simulink model "untitled"  (R2017b)
settings: Solver=VariableStepAuto  StartTime=0.0  StopTime=10.0  RelTol=1e-3
undefined symbols (not defined in the file): b_contact_RW, C_F_alpha, C_F_kappa, Cylinder, Dtheta0, epsilon, g, k_contact_RW, lengthRW, massRW, Parts_Lib, radiusRW, sigma, v0, X, xPla, Y, yPla, Z, zPla
libraries: nesl_utility x20, sm_lib x11, vrlib x6
settings Model: Creator=r_ahmed_afzal  LastModifiedBy=r_ahmed_afzal

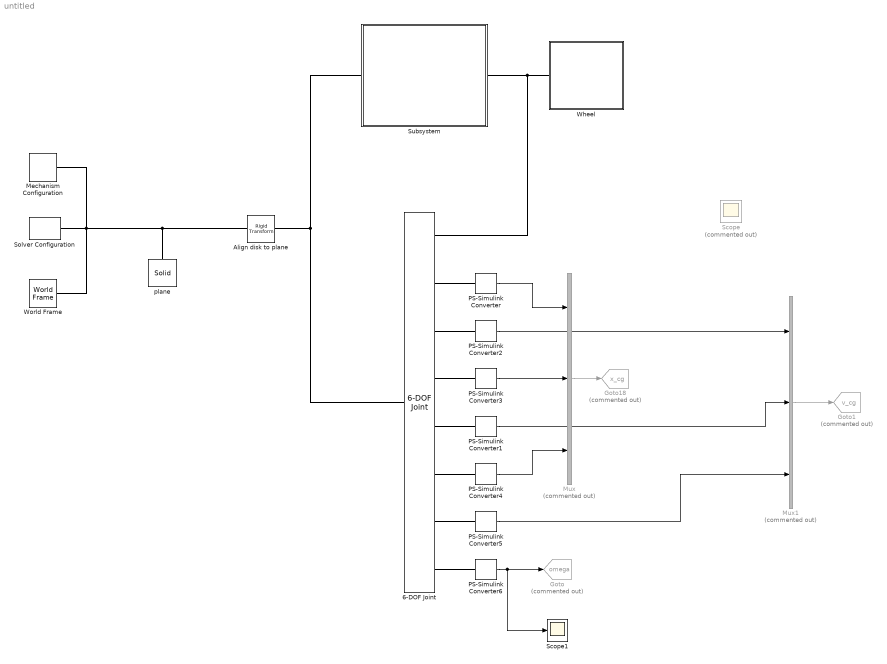
== system untitled ==
  6-DOF Joint : sm_lib/Joints/6-DOF Joint  SenseConstraintForce=off  SenseConstraintForceX=off  SenseConstraintForceY=off  SenseConstraintForceZ=off  SenseConstraintTorque=off  SenseConstraintTorqueX=off  SenseConstraintTorqueY=off  SenseConstraintTorqueZ=off  SenseTotalForce=off  SenseTotalForceX=off  SenseTotalForceY=off  SenseTotalForceZ=off  SenseTotalTorque=off  SenseTotalTorqueX=off  SenseTotalTorqueY=off  SenseTotalTorqueZ=off  CompositeWrenchDir=FollowerOnBase  CompositeWrenchFrame=BaseFrame  PxEquilibriumPosition=0  PxEquilibriumPositionUnits=m  PxSpringStiffness=0  PxSpringStiffnessUnits=N/m  PxDampingCoefficient=0  PxDampingCoefficientUnits=N/(m/s)  PxTorqueActuationMode=NoTorque  PxMotionActuationMode=ComputedMotion  PxSensePosition=on  PxSenseVelocity=on  PxSenseAcceleration=off  PxSenseTorqueForce=off  PxPositionTargetSpecify=on  PxPositionTargetPriority=High  PxPositionTargetValue=-xPla/2 + 0.1  PxPositionTargetValueUnits=m  PxVelocityTargetSpecify=off  PxVelocityTargetPriority=High  PxVelocityTargetValue=0  PxVelocityTargetValueUnits=m/s  PyEquilibriumPosition=0  PyEquilibriumPositionUnits=m  PySpringStiffness=0  PySpringStiffnessUnits=N/m  PyDampingCoefficient=0  PyDampingCoefficientUnits=N/(m/s)  PyTorqueActuationMode=NoTorque  PyMotionActuationMode=ComputedMotion  PySensePosition=on  PySenseVelocity=on  PySenseAcceleration=off  PySenseTorqueForce=off  PyPositionTargetSpecify=on  PyPositionTargetPriority=High  PyPositionTargetValue=radiusRW  PyPositionTargetValueUnits=m  PyVelocityTargetSpecify=off  PyVelocityTargetPriority=High  PyVelocityTargetValue=0  PyVelocityTargetValueUnits=m/s  PzEquilibriumPosition=0  PzEquilibriumPositionUnits=m  PzSpringStiffness=0  PzSpringStiffnessUnits=N/m  PzDampingCoefficient=0  PzDampingCoefficientUnits=N/(m/s)  PzTorqueActuationMode=NoTorque  PzMotionActuationMode=ComputedMotion  PzSensePosition=on  PzSenseVelocity=on  PzSenseAcceleration=off  PzSenseTorqueForce=off  PzPositionTargetSpecify=off  PzPositionTargetPriority=High  PzPositionTargetValue=0  PzPositionTargetValueUnits=m  PzVelocityTargetSpecify=off  PzVelocityTargetPriority=High  PzVelocityTargetValue=0  PzVelocityTargetValueUnits=m/s  SphDefPosRotationMethod=None  SphDefPosRotationAngleUnits=deg  SphDefPosRotationStandardAxis=+Z  SphDefPosRotationAngle=0.0  SphDefPosRotationArbitraryAxis=[0 0 1]  SphDefPosFollAlignAxisA=+X  SphDefPosBaseAlignAxisA=+Y  SphDefPosFollAlignAxisB=+Y  SphDefPosBaseAlignAxisB=+Z  SphDefPosRotationSequenceAxes=FollowerAxes  SphDefPosRotationSequence=XYX  SphDefPosRotationSequenceAngles=[0 0 0]  SphDefPosRotationSequenceAnglesUnits=deg  SphDefPosRotationMatrix=[1 0 0; 0 1 0; 0 0 1]  SphEqPosRotationMethod=None  SphEqPosRotationAngleUnits=deg  SphEqPosRotationStandardAxis=+Z  SphEqPosRotationAngle=0.0  SphEqPosRotationArbitraryAxis=[0 0 1]  SphEqPosFollAlignAxisA=+X  SphEqPosBaseAlignAxisA=+Y  SphEqPosFollAlignAxisB=+Y  SphEqPosBaseAlignAxisB=+Z  SphEqPosRotationSequenceAxes=FollowerAxes  SphEqPosRotationSequence=XYX  SphEqPosRotationSequenceAngles=[0 0 0]  SphEqPosRotationSequenceAnglesUnits=deg  SphEqPosRotationMatrix=[1 0 0; 0 1 0; 0 0 1]  SphSpringStiffness=0  SphSpringStiffnessUnits=N*m/deg  SphDampingCoefficient=0  SphDampingCoefficientUnits=N*m/(deg/s)  SphActuateTorqueX=off  SphActuateTorqueY=off  SphActuateTorqueZ=off  SphActuateTorque=off  SphTorqueActuationMode=NoTorque  SphMotionActuationMode=ComputedMotion  SphActuationFrame=BaseFrame  SphSensePosition=off  SphSenseVelocityX=off  SphSenseVelocityY=off  SphSenseVelocityZ=off  SphSenseVelocity=on  SphSenseAccelerationX=off  SphSenseAccelerationY=off  SphSenseAccelerationZ=off  SphSenseAcceleration=off  SphSenseTorqueX=off  SphSenseTorqueY=off  SphSenseTorqueZ=off  SphSenseTorqueForce=off  SphSensingFrame=FollowerFrame  SphPositionTargetRotationMethod=None  SphPositionTargetRotationAngleUnits=deg  SphPositionTargetRotationStandardAxis=+Z  SphPositionTargetRotationAngle=0.0  SphPositionTargetRotationArbitraryAxis=[0 0 1]  SphPositionTargetFollAlignAxisA=+X  SphPositionTargetBaseAlignAxisA=+Y  SphPositionTargetFollAlignAxisB=+Y  SphPositionTargetBaseAlignAxisB=+Z  SphPositionTargetRotationSequenceAxes=FollowerAxes  SphPositionTargetRotationSequence=XYX  SphPositionTargetRotationSequenceAngles=[0 0 0]  SphPositionTargetRotationSequenceAnglesUnits=deg  SphPositionTargetRotationMatrix=[1 0 0; 0 1 0; 0 0 1]  SphPositionTargetSpecify=off  SphPositionTargetPriority=High  SphVelocityTargetValue=[0 0 Dtheta0]  SphVelocityTargetValueUnits=rad/s  SphVelocityTargetSpecify=on  SphVelocityTargetPriority=High  SphVelocityTargetInFollowerFrame=on
  Align disk to plane : sm_lib/Frames and Transforms/Rigid Transform  TranslationMethod=None  TranslationStandardOffset=0  TranslationLengthUnit=m  TranslationStandardAxis=+Z  TranslationCartesianOffset=[0 0 0]  TranslationROffset=0  TranslationROffsetUnits=m  TranslationZOffset=0  TranslationZOffsetUnits=m  TranslationThetaOffset=0  TranslationThetaOffsetUnits=deg  RotationMethod=AlignedAxes  RotationAngleUnits=deg  RotationStandardAxis=-X  RotationAngle=90  RotationArbitraryAxis=[0 0 1]  FollAlignAxisA=+Y  BaseAlignAxisA=+Z  FollAlignAxisB=+X  BaseAlignAxisB=+X  RotationSequenceAxes=FollowerAxes  RotationSequence=XYX  RotationSequenceAngles=[0 0 0]  RotationSequenceAnglesUnits=deg  RotationMatrix=[1 0 0; 0 1 0; 0 0 1]
  Goto : Goto  Commented=on  GotoTag=omega  TagVisibility=global
  Goto1 : Goto  Commented=on  GotoTag=v_cg  TagVisibility=global
  Goto18 : Goto  Commented=on  GotoTag=x_cg  TagVisibility=global
  Mechanism Configuration : sm_lib/Utilities/Mechanism Configuration  UniformGravity=Constant  GravityVector=[0 0 -g]  GravityUnits=m/s^2  LinearizationDelta=0.001
  Mux : Mux  Commented=on  Inputs=3
  Mux1 : Mux  Commented=on  Inputs=3
  PS-Simulink Converter{,1..6} (7 alike) : nesl_utility/PS-Simulink Converter  PhysicalDomain=network_engine_domain  SubClassName=ps_output  LeftPortType=input  RightPortType=output  PseudoPeriodic=off  Frequencies=[]  Unit=1  AffineConversion=off
  Scope : Scope  Commented=on
  Scope1 : Scope
  Solver Configuration : nesl_utility/Solver Configuration  PhysicalDomain=network_engine_domain  SubClassName=solver  LeftPortType=input  RightPortType=generic  Accelerate=off  Tones=[]  Harmonics=[]  SimulateNoise=off  Profile=off  UseLocalSampling=off  EnableSwitchedLinearOptims=on  FrequencyDomain=off  UseCCode=off  RelTol=0.001  AbsTol=1e-06  MinStep=1e-09  ToWorkspace=off  RevertToSquareIcSolve=off  NumHomotopyIterations=100  PhasorMode=off  PhasorModeNumHarmonics=1  DoDC=off  ResidualTolerance=1e-09  UseLocalSolver=off  LocalSolverChoice=NE_BACKWARD_EULER_ADVANCER  LocalSolverSampleTime=0.001  DoFixedCost=off  MaxNonlinIter=3  MaxModeIter=2  LinearAlgebra=Sparse  DelaysMemoryBudget=1024  AutomaticFiltering=on  FilteringTimeConstant=0.001
  Subsystem : Subsystem
  Wheel : Subsystem  Tag=CustomStyle  AncestorBlock=Parts_Lib/Cylinder  mask(Solid Cylinder with Markings){cyl_radius=radiusRW, cyl_length=lengthRW, cyl_density=1000, cyl_color=blue, cyl_opacity=1, cyl_color_custom=[0.7920    0.9900    0.9900], mark_radius=[0.75 0.5], mark_len_factor=1.01, mark_angle=60, mark_color=purple, mark_opacity=1}
      mask prompts: cyl_radius "Radius (m)"; cyl_length "Length (m)"; cyl_density "Density (kg/m^3)"; cyl_color "Color"; cyl_opacity "Opacity (0-1)"; cyl_color_custom "Custom Color (rgb)"; mark_radius "Outer, inner radius (% of cylinder radius)"; mark_len_factor "Length (factor of cylinder length)"; mark_angle "Sweep angle (deg)"; mark_color "Color"; mark_opacity "Opacity (0-1)"
      mask init:
      | curblk = gcb;
      | if strcmp(get_param(curblk,'cyl_color'),'red')
      |     set_param([curblk '/Cylinder'],'GraphicDiffuseColor','[0.8 0.0 0.2]');
      |     set_param(curblk,'BackGroundColor','[0.901961, 0.396078, 0.396078]');
      | elseif strcmp(get_param(gcb,'cyl_color'),'blue')
      |     set_param([curblk '/Cylinder'],'GraphicDiffuseColor','[0.0 0.5 0.7]');
      |     set_param(curblk,'BackGroundColor','[0.541176, 0.698039, 0.901961]');
      | elseif strcmp(get_param(gcb,'cyl_color'),'yellow')
      |     set_param([curblk '/Cylinder'],'GraphicDiffuseColor','[1.0 1.0 0.0]');
      |     set_param(curblk,'BackGroundColor','[0.905882, 0.890196, 0.392157]');
      | elseif strcmp(get_param(gcb,'cyl_color'),'gray')
      |     set_param([curblk '/Cylinder'],'GraphicDiffuseColor','[1.0 1.0 1.0]*0.6');
      |     set_param(curblk,'BackGroundColor','[0.6 0.6 0.6]');
      | elseif strcmp(get_param(gcb,'cyl_color'),'custom')
      |     set_param([curblk '/Cylinder'],'GraphicDiffuseColor',get_param(curblk,'cyl_color_custom'));
      |     set_param(curblk,'BackGroundColor','[1 1 1]');
      | end
      | 
      | if strcmp(get_param(curblk,'mark_color'),'purple')
      |     set_param([curblk '/Vis1'],'GraphicDiffuseColor','[0.4 0.0 0.4]');
      |     set_param([curblk '/Vis2'],'GraphicDiffuseColor','[0.4 0.0 0.4]');
      | elseif strcmp(get_param(gcb,'mark_color'),'green')
      |     set_param([curblk '/Vis1'],'GraphicDiffuseColor','[0.0 0.8 0.0]');
      |     set_param([curblk '/Vis2'],'GraphicDiffuseColor','[0.0 0.8 0.0]');
      | elseif strcmp(get_param(gcb,'mark_color'),'orange')
      |     set_param([curblk '/Vis1'],'GraphicDiffuseColor','[1.0 0.6 0.0]');
      |     set_param([curblk '/Vis2'],'GraphicDiffuseColor','[1.0 0.6 0.0]');
      | elseif strcmp(get_param(gcb,'mark_color'),'black')
      |     set_param([curblk '/Vis1'],'GraphicDiffuseColor','[0.0 0.0 0.0]');
      |     set_param([curblk '/Vis2'],'GraphicDiffuseColor','[0.0 0.0 0.0]');
      | end
      | 
      | clear curblk
      mask TypeOptions cyl_color: red | gray | yellow | blue | custom
      mask Callback cyl_color:
      | maskObj = Simulink.Mask.get(gcb);
      | clr_h = maskObj.getParameter('cyl_color_custom');
      | if strcmp(get_param(gcb,'cyl_color'),'custom')
      |     clr_h.Visible = 'on';
      | else
      |     clr_h.Visible = 'off';
      | end
      mask TypeOptions mark_color: purple | green | orange | black
      mask DialogControl Container4 Prompt: Cylinder
      mask DialogControl Container7 Prompt: Markings
  World Frame : sm_lib/Frames and Transforms/World Frame
  plane : sm_lib/Body Elements/Solid  InertiaType=CalculateFromGeometry  Mass=1  MassUnits=kg  CenterOfMass=[0 0 0]  CenterOfMassUnits=m  MomentsOfInertia=[1 1 1]  MomentsOfInertiaUnits=kg*m^2  ProductsOfInertia=[1 1 1]  ProductsOfInertiaUnits=kg*m^2  DensityBased=on  Density=1000  DensityUnits=kg/m^3  DoExposeReferenceFrame=on  SerializedFrames=<Frames/>  GraphicType=FromGeometry  MarkerShape=Sphere  MarkerSize=10  GraphicVisPropType=SimpleVisualProperties  GraphicDiffuseColor=[0.5 0.5 0.5]  GraphicSpecularColor=[0.5 0.5 0.5 1.0]  GraphicAmbientColor=[0.15 0.15 0.15 1.0]  GraphicEmissiveColor=[0.0 0.0 0.0 1.0]  GraphicShininess=75  GraphicOpacity=0.5  GeometryShape=Brick  RectangleSize=[1 1]  RectangleSizeUnits=m  BrickDimensions=[xPla yPla zPla]  BrickDimensionUnits=m  CylinderRadius=1  CylinderRadiusUnits=m  CylinderLength=1  CylinderLengthUnits=m  SphereRadius=1  SphereRadiusUnits=m  EllipsoidRadii=[1 1 1]  EllipsoidRadiiUnits=m  ExtrusionCrossSection=[1 1; -1 1; -1 -1; 1 -1]  ExtrusionCrossSectionUnits=m  ExtrusionLength=1  ExtrusionLengthUnits=m  PolygonNumSides=3  PolygonOuterRadius=1  PolygonOuterRadiusUnits=m  ExtGeomFileType=STEP  ExtGeomFileUnits=m  RevolutionCrossSection=[1 1; 1 -1; 2 -1; 2 1]  RevolutionCrossSectionUnits=m  RevolutionExtent=Full  RevolutionAngle=180  RevolutionAngleUnits=deg
  wires:
  PS-Simulink Converter6/1 -> Scope1/1, Goto/1
  PS-Simulink Converter/1 -> Mux/1
  PS-Simulink Converter3/1 -> Mux/2
  PS-Simulink Converter4/1 -> Mux/3
  Mux/1 -> Goto18/1
  PS-Simulink Converter2/1 -> Mux1/1
  PS-Simulink Converter1/1 -> Mux1/2
  PS-Simulink Converter5/1 -> Mux1/3
  Mux1/1 -> Goto1/1
  connections:
  plane/RConn1 -- Mechanism Configuration/RConn1 -- Solver Configuration/RConn1 -- World Frame/RConn1 -- Align disk to plane/LConn1
  6-DOF Joint/LConn1 -- Subsystem/LConn1 -- Align disk to plane/RConn1
  Wheel/LConn1 -- 6-DOF Joint/RConn1 -- Subsystem/RConn1
  PS-Simulink Converter/LConn1 -- 6-DOF Joint/RConn2
  6-DOF Joint/RConn3 -- PS-Simulink Converter2/LConn1
  6-DOF Joint/RConn4 -- PS-Simulink Converter3/LConn1
  6-DOF Joint/RConn5 -- PS-Simulink Converter1/LConn1
  PS-Simulink Converter4/LConn1 -- 6-DOF Joint/RConn6
  PS-Simulink Converter5/LConn1 -- 6-DOF Joint/RConn7
  PS-Simulink Converter6/LConn1 -- 6-DOF Joint/RConn8

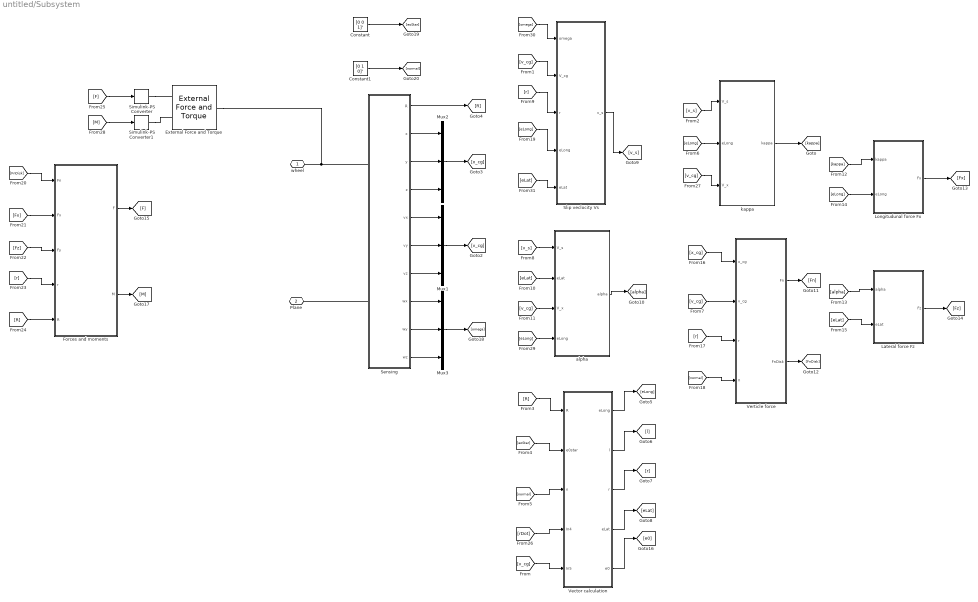
== system untitled/Subsystem ==
  Constant : Constant  Value=[0 0 1]'
  Constant1 : Constant  Value=[0 1 0]'
  External Force and Torque : sm_lib/Forces and Torques/External Force and Torque  ForceResolutionFrame=AttachedFrame  EnableForceX=off  EnableForceY=off  EnableForceZ=off  EnableForce=on  TorqueResolutionFrame=AttachedFrame  EnableTorqueX=off  EnableTorqueY=off  EnableTorqueZ=off  EnableTorque=on
  Forces and moments : Subsystem
  Lateral force Fz : Subsystem
  Longitudunal force Fx : Subsystem
  Mux1 : Mux  Inputs=3
  Mux2 : Mux  Inputs=3
  Mux3 : Mux  Inputs=3
  Sensing : Subsystem
  Simulink-PS Converter : nesl_utility/Simulink-PS Converter  PhysicalDomain=network_engine_domain  SubClassName=ps_input  LeftPortType=input  RightPortType=output  PseudoPeriodic=off  Frequencies=[]  NoiseDistribution=none  NoiseParameters=[]  Unit=1  AffineConversion=off  FilteringAndDerivatives=provide  SimscapeFilterOrder=1  InputFilterTimeConstant=0.001  UdotUserProvided=0
  Simulink-PS Converter1 : nesl_utility/Simulink-PS Converter  PhysicalDomain=network_engine_domain  SubClassName=ps_input  LeftPortType=input  RightPortType=output  PseudoPeriodic=off  Frequencies=[]  NoiseDistribution=none  NoiseParameters=[]  Unit=1  AffineConversion=off  FilteringAndDerivatives=provide  SimscapeFilterOrder=1  InputFilterTimeConstant=0.001  UdotUserProvided=0
  Slip veclocity Vs : Subsystem
  Vector calculation : Subsystem
  Verticle force : Subsystem
  alpha : Subsystem
  kappa : Subsystem
  wheel : PMIOPort  Port=1  Side=Right
  Plane : PMIOPort  Port=2  Side=Left
  wires:
  Mux1/1 -> [v_cg]
  Sensing/6(vy) -> Mux1/2
  Sensing/2(x) -> Mux2/1
  Sensing/4(z) -> Mux2/3
  Sensing/9(wy) -> Mux3/2
  Sensing/1(R) -> [R]
  Sensing/7(vz) -> Mux1/3
  Mux2/1 -> [x_cg]
  Sensing/8(wx) -> Mux3/1
  Sensing/5(vx) -> Mux1/1
  Sensing/3(y) -> Mux2/2
  Slip veclocity Vs/1(v_s) -> [v_s]
  [omega] -> Slip veclocity Vs/1(omega)
  [v_s] -> kappa/1(V_s)
  [rDot] -> Vector calculation/4(In4)
  [eoStar] -> Vector calculation/2(e0star)
  Vector calculation/5(e0) -> [e0]
  Vector calculation/3(r) -> [r]
  [normal] -> Vector calculation/3(n)
  Vector calculation/2(l) -> [l]
  Vector calculation/4(eLat) -> [eLat]
  [R] -> Vector calculation/1(R)
  Vector calculation/1(eLong) -> [eLong]
  [eLong] -> kappa/2(eLong)
  [v_cg] -> kappa/3(V_x)
  [eLat] -> alpha/2(eLat)
  [v_s] -> alpha/1(V_s)
  [v_cg] -> alpha/3(V_x)
  kappa/1(kappa) -> [kappa]
  alpha/1(alpha) -> [alpha]
  [kappa] -> Longitudunal force Fx/1(kappa)
  [alpha] -> Lateral force Fz/1(alpha)
  [eLong] -> Longitudunal force Fx/2(eLong)
  [eLat] -> Lateral force Fz/2(eLat)
  [normal] -> Verticle force/4(n)
  [r] -> Verticle force/3(r)
  Verticle force/2(FnDisk) -> [FnDisk]
  Verticle force/1(Fn) -> [Fn]
  [v_cg] -> Verticle force/2(v_cg)
  [x_cg] -> Verticle force/1(x_cg)
  [FnDisk] -> Forces and moments/1(Fn)
  Longitudunal force Fx/1(Fx) -> [Fx]
  Lateral force Fz/1(Fz) -> [Fz]
  [Fx] -> Forces and moments/2(Fx)
  [Fz] -> Forces and moments/3(Fy)
  [r] -> Forces and moments/4(r)
  [R] -> Forces and moments/5(R)
  Forces and moments/1(F) -> [F]
  Forces and moments/2(M) -> [M]
  [F] -> Simulink-PS Converter/1
  [M] -> Simulink-PS Converter1/1
  Constant/1 -> [eoStar]
  Constant1/1 -> [normal]
  [v_cg] -> Vector calculation/5(In5)
  [eLong] -> alpha/4(eLong)
  [eLong] -> Slip veclocity Vs/4(eLong)
  [eLat] -> Slip veclocity Vs/5(eLat)
  [r] -> Slip veclocity Vs/3(r)
  Sensing/10(wz) -> Mux3/3
  Mux3/1 -> [omega]
  [v_cg] -> Slip veclocity Vs/2(V_cg)
  connections:
  Sensing/LConn1 -- External Force and Torque/RConn1 -- wheel/RConn1
  Sensing/LConn2 -- Plane/RConn1
  Simulink-PS Converter/RConn1 -- External Force and Torque/LConn1
  Simulink-PS Converter1/RConn1 -- External Force and Torque/LConn2

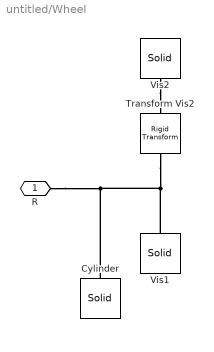
== system untitled/Wheel ==
  Cylinder : sm_lib/Body Elements/Solid  InertiaType=Custom  Mass=massRW  MassUnits=kg  CenterOfMass=[0 0 0]  CenterOfMassUnits=m  MomentsOfInertia=momentInertiaRW  MomentsOfInertiaUnits=kg*m^2  ProductsOfInertia=[0 0 0]  ProductsOfInertiaUnits=kg*m^2  DensityBased=on  Density=cyl_density  DensityUnits=kg/(m^3)  DoExposeReferenceFrame=on  SerializedFrames=<Frames/>  GraphicType=FromGeometry  MarkerShape=Sphere  MarkerSize=10  MarkerSizeUnits=m  GraphicVisPropType=SimpleVisualProperties  GraphicDiffuseColor=[0.0 0.5 0.7]  GraphicSpecularColor=[0.5 0.5 0.5 1.0]  GraphicAmbientColor=[0.15 0.15 0.15 1.0]  GraphicEmissiveColor=[0.0 0.0 0.0 1.0]  GraphicShininess=75  GraphicOpacity=cyl_opacity  GeometryShape=Cylinder  RectangleSize=[1 1]  RectangleSizeUnits=m  BrickDimensions=[1 1 1]  BrickDimensionUnits=m  CylinderRadius=cyl_radius  CylinderRadiusUnits=m  CylinderLength=cyl_length  CylinderLengthUnits=m  SphereRadius=1  SphereRadiusUnits=m  EllipsoidRadii=[1 1 1]  EllipsoidRadiiUnits=m  ExtrusionCrossSection=[1 1; -1 1; -1 -1; 1 -1]  ExtrusionCrossSectionUnits=m  ExtrusionLength=1  ExtrusionLengthUnits=m  PolygonNumSides=3  PolygonOuterRadius=1  PolygonOuterRadiusUnits=m  ExtGeomFileType=STL  ExtGeomFileUnits=m  RevolutionCrossSection=[1 1; 1 -1; 2 -1; 2 1]  RevolutionCrossSectionUnits=m  RevolutionExtent=Full  RevolutionAngle=180  RevolutionAngleUnits=deg
  Transform Vis2 : sm_lib/Frames and Transforms/Rigid Transform  TranslationMethod=None  TranslationStandardOffset=0  TranslationLengthUnit=m  TranslationStandardAxis=+Z  TranslationCartesianOffset=[0 0 0]  TranslationROffset=0  TranslationROffsetUnits=m  TranslationZOffset=0  TranslationZOffsetUnits=m  TranslationThetaOffset=0  TranslationThetaOffsetUnits=deg  RotationMethod=StandardAxis  RotationAngleUnits=deg  RotationStandardAxis=+Y  RotationAngle=180  RotationArbitraryAxis=[0 0 1]  FollAlignAxisA=+X  BaseAlignAxisA=+Y  FollAlignAxisB=+Y  BaseAlignAxisB=+Z  RotationSequenceAxes=FollowerAxes  RotationSequence=XYX  RotationSequenceAngles=[0 0 0]  RotationSequenceAnglesUnits=deg  RotationMatrix=[1 0 0; 0 1 0; 0 0 1]
  Vis1 : sm_lib/Body Elements/Solid  InertiaType=CalculateFromGeometry  Mass=1  MassUnits=kg  CenterOfMass=[0 0 0]  CenterOfMassUnits=m  MomentsOfInertia=[1 1 1]  MomentsOfInertiaUnits=kg*m^2  ProductsOfInertia=[0 0 0]  ProductsOfInertiaUnits=kg*m^2  DensityBased=on  Density=1e-3  DensityUnits=kg/(m^3)  DoExposeReferenceFrame=on  SerializedFrames=<Frames/>  GraphicType=FromGeometry  MarkerShape=Sphere  MarkerSize=10  MarkerSizeUnits=m  GraphicVisPropType=SimpleVisualProperties  GraphicDiffuseColor=[0.4 0.0 0.4]  GraphicSpecularColor=[0.5 0.5 0.5 1.0]  GraphicAmbientColor=[0.15 0.15 0.15 1.0]  GraphicEmissiveColor=[0.0 0.0 0.0 1.0]  GraphicShininess=75  GraphicOpacity=mark_opacity  GeometryShape=GeneralSolidOfRevolution  RectangleSize=[1 1]  RectangleSizeUnits=m  BrickDimensions=[1 1 1]  BrickDimensionUnits=m  CylinderRadius=0.1  CylinderRadiusUnits=m  CylinderLength=0.01  CylinderLengthUnits=m  SphereRadius=1  SphereRadiusUnits=m  EllipsoidRadii=[1 1 1]  EllipsoidRadiiUnits=m  ExtrusionCrossSection=[1 1; -1 1; -1 -1; 1 -1]  ExtrusionCrossSectionUnits=m  ExtrusionLength=1  ExtrusionLengthUnits=m  PolygonNumSides=3  PolygonOuterRadius=1  PolygonOuterRadiusUnits=m  ExtGeomFileType=STL  ExtGeomFileUnits=m  RevolutionCrossSection=[cyl_radius*mark_radius(1) cyl_length/2*mark_len_factor; cyl_radius*mark_radius(2) cyl_length/2*mark_len_factor; cyl_radius*mark_radius(2) -cyl_length/2*mark_len_factor; cyl_radius*mark_radius(1) -cyl_length/2*mark_len_factor]  RevolutionCrossSectionUnits=m  RevolutionExtent=Custom  RevolutionAngle=mark_angle  RevolutionAngleUnits=deg
  Vis2 : sm_lib/Body Elements/Solid  InertiaType=CalculateFromGeometry  Mass=1  MassUnits=kg  CenterOfMass=[0 0 0]  CenterOfMassUnits=m  MomentsOfInertia=[1 1 1]  MomentsOfInertiaUnits=kg*m^2  ProductsOfInertia=[0 0 0]  ProductsOfInertiaUnits=kg*m^2  DensityBased=on  Density=1e-3  DensityUnits=kg/(m^3)  DoExposeReferenceFrame=on  SerializedFrames=<Frames/>  GraphicType=FromGeometry  MarkerShape=Sphere  MarkerSize=10  MarkerSizeUnits=m  GraphicVisPropType=SimpleVisualProperties  GraphicDiffuseColor=[0.4 0.0 0.4]  GraphicSpecularColor=[0.5 0.5 0.5 1.0]  GraphicAmbientColor=[0.15 0.15 0.15 1.0]  GraphicEmissiveColor=[0.0 0.0 0.0 1.0]  GraphicShininess=75  GraphicOpacity=mark_opacity  GeometryShape=GeneralSolidOfRevolution  RectangleSize=[1 1]  RectangleSizeUnits=m  BrickDimensions=[1 1 1]  BrickDimensionUnits=m  CylinderRadius=0.1  CylinderRadiusUnits=m  CylinderLength=0.01  CylinderLengthUnits=m  SphereRadius=1  SphereRadiusUnits=m  EllipsoidRadii=[1 1 1]  EllipsoidRadiiUnits=m  ExtrusionCrossSection=[1 1; -1 1; -1 -1; 1 -1]  ExtrusionCrossSectionUnits=m  ExtrusionLength=1  ExtrusionLengthUnits=m  PolygonNumSides=3  PolygonOuterRadius=1  PolygonOuterRadiusUnits=m  ExtGeomFileType=STL  ExtGeomFileUnits=m  RevolutionCrossSection=[cyl_radius*mark_radius(1) cyl_length/2*mark_len_factor; cyl_radius*mark_radius(2) cyl_length/2*mark_len_factor; cyl_radius*mark_radius(2) -cyl_length/2*mark_len_factor; cyl_radius*mark_radius(1) -cyl_length/2*mark_len_factor]  RevolutionCrossSectionUnits=m  RevolutionExtent=Custom  RevolutionAngle=mark_angle  RevolutionAngleUnits=deg
  R : PMIOPort  Port=1  Side=Left
  connections:
  Vis2/RConn1 -- Transform Vis2/RConn1
  Vis1/RConn1 -- Transform Vis2/LConn1 -- Cylinder/RConn1 -- R/RConn1

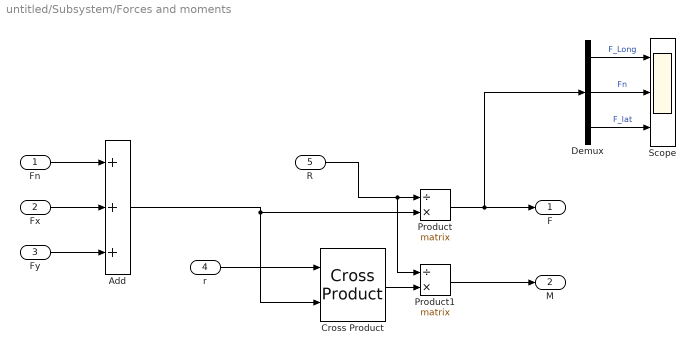
== system untitled/Subsystem/Forces and moments ==
  Fn : Inport
  Fx : Inport  Port=2
  Fy : Inport  Port=3
  r : Inport  Port=4
  R : Inport  Port=5
  Add : Sum  Inputs=3
  Cross Product : vrlib/Utilities/Cross Product
      settings: SourceProductBaseCode=VR
  Demux : Demux  Outputs=3
  Product : Product  Inputs=/*  Multiplication=Matrix(*)
  Product1 : Product  Inputs=/*  Multiplication=Matrix(*)
  Scope : Scope  NumInputPorts=3
  F : Outport
  M : Outport  Port=2
  wires:
  Fn/1 -> Add/1
  Fy/1 -> Add/3
  Product/1 -> Demux/1, F/1
  R/1 -> Product1/1, Product/1
  Add/1 -> Cross Product/2, Product/2
  Fx/1 -> Add/2
  Cross Product/1 -> Product1/2
  Product1/1 -> M/1
  Demux/3 -> Scope/3  "F_lat"
  Demux/2 -> Scope/2  "Fn"
  Demux/1 -> Scope/1  "F_Long"
  r/1 -> Cross Product/1

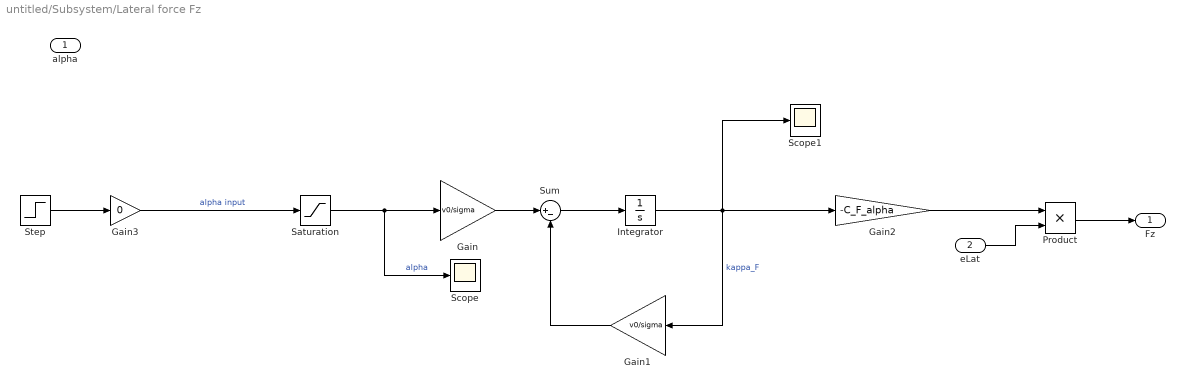
== system untitled/Subsystem/Lateral force Fz ==
  alpha : Inport
  eLat : Inport  Port=2
  Gain : Gain  Gain=v0/sigma
  Gain1 : Gain  Gain=v0/sigma
  Gain2 : Gain  Gain=-C_F_alpha
  Gain3 : Gain  Gain=0
  Integrator : Integrator
  Product : Product
  Saturation : Saturate  UpperLimit=0  LowerLimit=-1e0
  Scope : Scope
  Scope1 : Scope
  Step : Step  Time=0  SampleTime=0
  Sum : Sum  Inputs=|+-
  Fz : Outport
  wires:
  Gain/1 -> Sum/1
  Sum/1 -> Integrator/1
  Integrator/1 -> Scope1/1, Gain1/1, Gain2/1  "kappa_F"
  Gain1/1 -> Sum/2
  Gain2/1 -> Product/1
  eLat/1 -> Product/2
  Saturation/1 -> Scope/1, Gain/1  "alpha"
  Step/1 -> Gain3/1
  Gain3/1 -> Saturation/1  "alpha input"
  Product/1 -> Fz/1

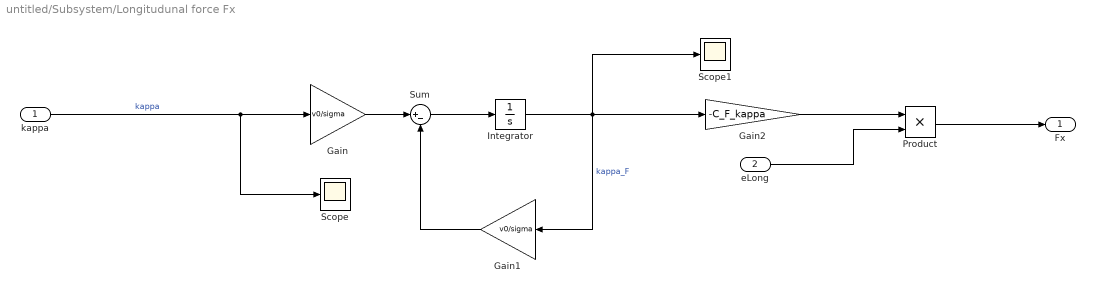
== system untitled/Subsystem/Longitudunal force Fx ==
  kappa : Inport
  eLong : Inport  Port=2
  Gain : Gain  Gain=v0/sigma
  Gain1 : Gain  Gain=v0/sigma
  Gain2 : Gain  Gain=-C_F_kappa
  Integrator : Integrator
  Product : Product
  Scope : Scope
  Scope1 : Scope
  Sum : Sum  Inputs=|+-
  Fx : Outport
  wires:
  Gain/1 -> Sum/1
  Sum/1 -> Integrator/1
  Integrator/1 -> Scope1/1, Gain1/1, Gain2/1  "kappa_F"
  Gain1/1 -> Sum/2
  Gain2/1 -> Product/1
  eLong/1 -> Product/2
  Product/1 -> Fx/1
  kappa/1 -> Scope/1, Gain/1  "kappa"

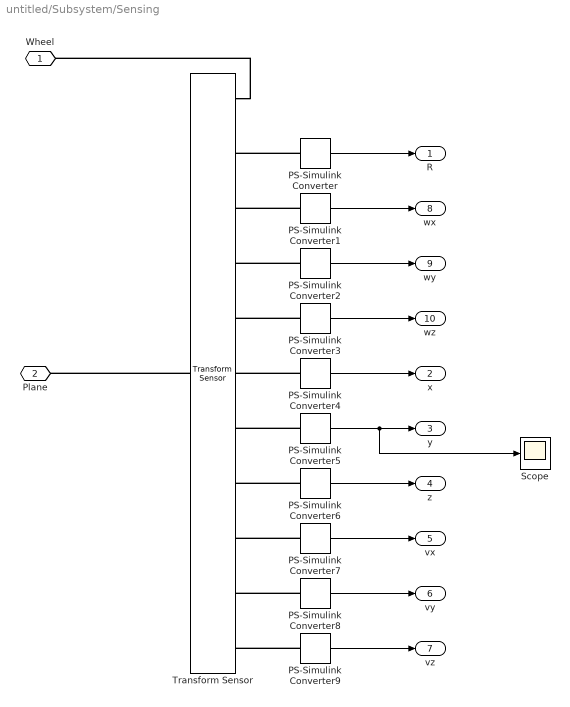
== system untitled/Subsystem/Sensing ==
  PS-Simulink Converter{,1..9} (10 alike) : nesl_utility/PS-Simulink Converter  PhysicalDomain=network_engine_domain  SubClassName=ps_output  LeftPortType=input  RightPortType=output  PseudoPeriodic=off  Frequencies=[]  Unit=1  AffineConversion=off
  Scope : Scope
  Transform Sensor : sm_lib/Frames and Transforms/Transform Sensor  MeasurementFrame=Base  SenseAngle=off  SenseAxis=off  SenseAngle1=off  SenseAngle2=off  SenseAngle3=off  SenseQ=off  SenseR=on  SenseOmegaX=on  SenseOmegaY=on  SenseOmegaZ=on  SenseOmega1=off  SenseOmega2=off  SenseOmega3=off  SenseQDot=off  SenseRDot=off  SenseAlphaX=off  SenseAlphaY=off  SenseAlphaZ=off  SenseAlpha1=off  SenseAlpha2=off  SenseAlpha3=off  SenseQDDot=off  SenseRDDot=off  SenseX=on  SenseY=on  SenseZ=on  SenseRad=off  SenseAzim=off  SenseDist=off  SenseInc=off  SenseXDot=on  SenseYDot=on  SenseZDot=on  SenseRadDot=off  SenseAzimDot=off  SenseDistDot=off  SenseIncDot=off  SenseXDDot=off  SenseYDDot=off  SenseZDDot=off  SenseRadDDot=off  SenseAzimDDot=off  SenseDistDDot=off  SenseIncDDot=off
  Wheel : PMIOPort  Port=1  Side=Left
  Plane : PMIOPort  Port=2  Side=Left
  R : Outport
  x : Outport  Port=2
  y : Outport  Port=3
  z : Outport  Port=4
  vx : Outport  Port=5
  vy : Outport  Port=6
  vz : Outport  Port=7
  wx : Outport  Port=8
  wy : Outport  Port=9
  wz : Outport  Port=10
  wires:
  PS-Simulink Converter2/1 -> wy/1
  PS-Simulink Converter8/1 -> vy/1
  PS-Simulink Converter9/1 -> vz/1
  PS-Simulink Converter1/1 -> wx/1
  PS-Simulink Converter4/1 -> x/1
  PS-Simulink Converter7/1 -> vx/1
  PS-Simulink Converter3/1 -> wz/1
  PS-Simulink Converter5/1 -> Scope/1, y/1
  PS-Simulink Converter6/1 -> z/1
  PS-Simulink Converter/1 -> R/1
  connections:
  PS-Simulink Converter1/LConn1 -- Transform Sensor/RConn3
  PS-Simulink Converter4/LConn1 -- Transform Sensor/RConn6
  PS-Simulink Converter3/LConn1 -- Transform Sensor/RConn5
  PS-Simulink Converter9/LConn1 -- Transform Sensor/RConn11
  PS-Simulink Converter2/LConn1 -- Transform Sensor/RConn4
  PS-Simulink Converter6/LConn1 -- Transform Sensor/RConn8
  PS-Simulink Converter/LConn1 -- Transform Sensor/RConn2
  Transform Sensor/LConn1 -- Plane/RConn1
  Transform Sensor/RConn1 -- Wheel/RConn1
  PS-Simulink Converter5/LConn1 -- Transform Sensor/RConn7
  PS-Simulink Converter7/LConn1 -- Transform Sensor/RConn9
  PS-Simulink Converter8/LConn1 -- Transform Sensor/RConn10

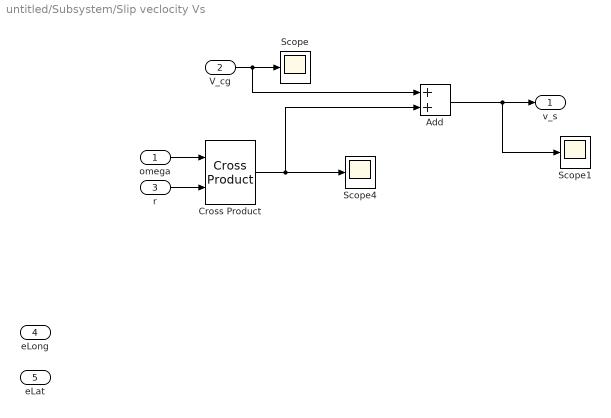
== system untitled/Subsystem/Slip veclocity Vs ==
  omega : Inport
  V_cg : Inport  Port=2
  r : Inport  Port=3
  eLong : Inport  Port=4
  eLat : Inport  Port=5
  Add : Sum
  Cross Product : vrlib/Utilities/Cross Product
      settings: SourceProductBaseCode=VR
  Scope : Scope
  Scope1 : Scope
  Scope4 : Scope
  v_s : Outport
  wires:
  Cross Product/1 -> Add/2, Scope4/1
  r/1 -> Cross Product/2
  omega/1 -> Cross Product/1
  V_cg/1 -> Add/1, Scope/1
  Add/1 -> Scope1/1, v_s/1

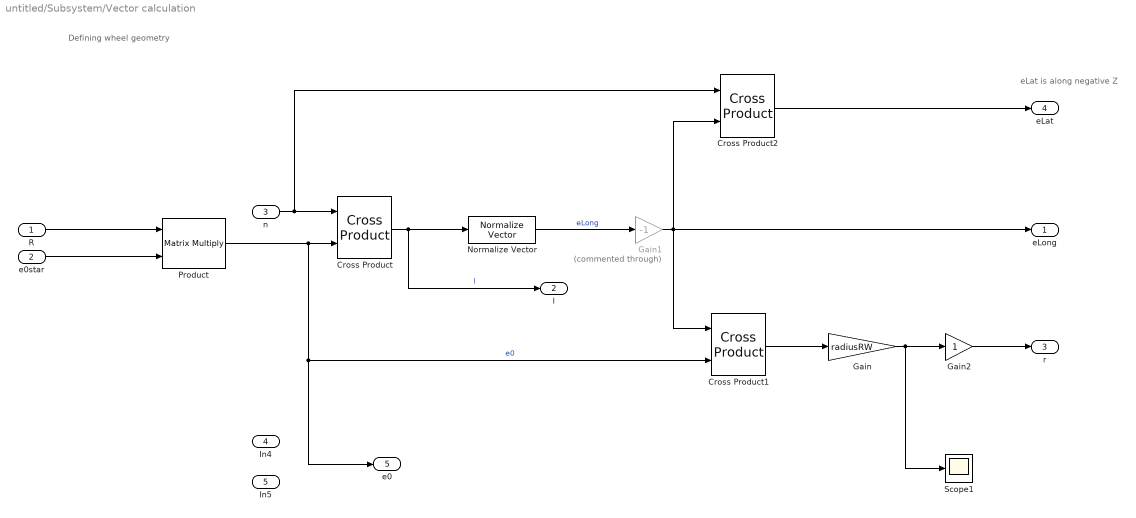
== system untitled/Subsystem/Vector calculation ==
  note: Defining wheel geometry
  note: eLat is along
      | negative Z
  R : Inport
  e0star : Inport  Port=2
  n : Inport  Port=3
  In4 : Inport  Port=4
  In5 : Inport  Port=5
  Cross Product : vrlib/Utilities/Cross Product
      settings: SourceProductBaseCode=VR
  Cross Product1 : vrlib/Utilities/Cross Product
      settings: SourceProductBaseCode=VR
  Cross Product2 : vrlib/Utilities/Cross Product
      settings: SourceProductBaseCode=VR
  Gain : Gain  Gain=radiusRW
  Gain1 : Gain  Commented=through  Gain=-1
  Gain2 : Gain
  Normalize Vector : vrlib/Utilities/Normalize Vector  maxzero=0
      settings: SourceProductName=Simulink 3D Animation  SourceProductBaseCode=VR
  Product : Product  Multiplication=Matrix(*)
  Scope1 : Scope
  eLong : Outport
  l : Outport  Port=2
  r : Outport  Port=3
  eLat : Outport  Port=4
  e0 : Outport  Port=5
  wires:
  R/1 -> Product/1
  e0star/1 -> Product/2
  Product/1 -> Cross Product1/2, e0/1, Cross Product/2  "e0"
  n/1 -> Cross Product2/1, Cross Product/1
  Cross Product/1 -> l/1, Normalize Vector/1  "l"
  Normalize Vector/1 -> Gain1/1  "eLong"
  Cross Product1/1 -> Gain/1
  Gain/1 -> Scope1/1, Gain2/1
  Cross Product2/1 -> eLat/1
  Gain1/1 -> eLong/1, Cross Product2/2, Cross Product1/1
  Gain2/1 -> r/1

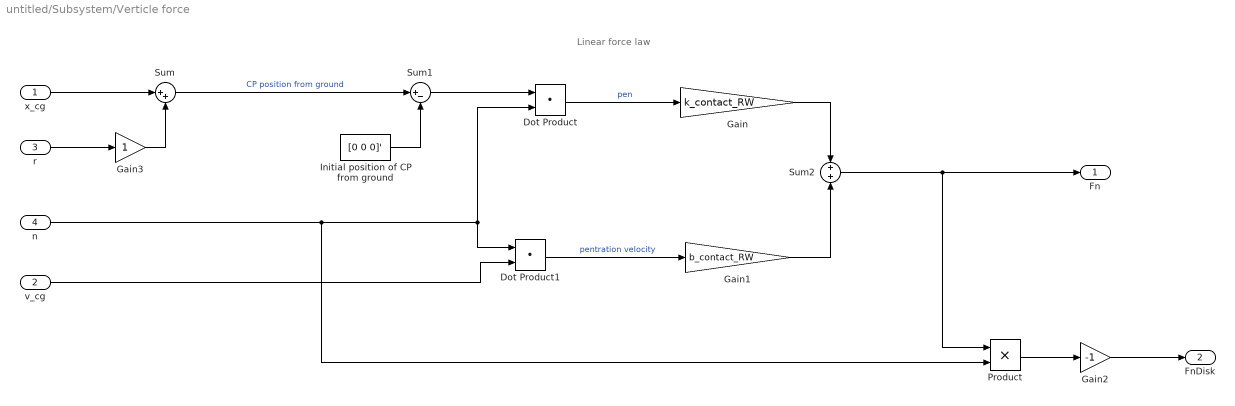
== system untitled/Subsystem/Verticle force ==
  note: Linear force law
  x_cg : Inport
  v_cg : Inport  Port=2
  r : Inport  Port=3
  n : Inport  Port=4
  Dot Product : DotProduct  InputSameDT=on  OutDataTypeStr=Inherit: Inherit via internal rule
  Dot Product1 : DotProduct  InputSameDT=on  OutDataTypeStr=Inherit: Inherit via internal rule
  Gain : Gain  Gain=k_contact_RW
  Gain1 : Gain  Gain=b_contact_RW
  Gain2 : Gain  Gain=-1
  Gain3 : Gain
  Initial position of CP from ground : Constant  Value=[0 0 0]'
  Product : Product
  Sum : Sum  Inputs=|++
  Sum1 : Sum  Inputs=|+-
  Sum2 : Sum
  Fn : Outport
  FnDisk : Outport  Port=2
  wires:
  x_cg/1 -> Sum/1
  Sum/1 -> Sum1/1  "CP position from ground"
  Initial position of CP from ground/1 -> Sum1/2
  Sum1/1 -> Dot Product/1
  Dot Product/1 -> Gain/1  "pen"
  v_cg/1 -> Dot Product1/2
  Dot Product1/1 -> Gain1/1  "pentration velocity"
  Gain1/1 -> Sum2/2
  Sum2/1 -> Product/1, Fn/1
  Product/1 -> Gain2/1
  n/1 -> Product/2, Dot Product1/1, Dot Product/2
  Gain/1 -> Sum2/1
  r/1 -> Gain3/1
  Gain3/1 -> Sum/2
  Gain2/1 -> FnDisk/1

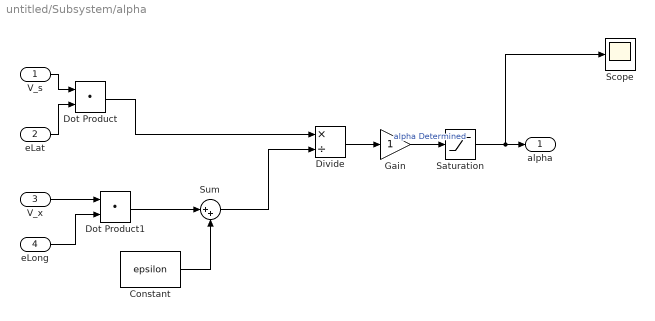
== system untitled/Subsystem/alpha ==
  V_s : Inport
  eLat : Inport  Port=2
  V_x : Inport  Port=3
  eLong : Inport  Port=4
  Constant : Constant  Value=epsilon
  Divide : Product  Inputs=*/
  Dot Product : DotProduct  InputSameDT=on  OutDataTypeStr=Inherit: Inherit via internal rule
  Dot Product1 : DotProduct  InputSameDT=on  OutDataTypeStr=Inherit: Inherit via internal rule
  Gain : Gain
  Saturation : Saturate  UpperLimit=0  LowerLimit=-1e0
  Scope : Scope
  Sum : Sum  Inputs=|++
  alpha : Outport
  wires:
  V_s/1 -> Dot Product/1
  eLat/1 -> Dot Product/2
  Dot Product/1 -> Divide/1
  V_x/1 -> Dot Product1/1
  Divide/1 -> Gain/1
  Gain/1 -> Saturation/1  "alpha Determined"
  Dot Product1/1 -> Sum/1
  Constant/1 -> Sum/2
  Sum/1 -> Divide/2
  eLong/1 -> Dot Product1/2
  Saturation/1 -> Scope/1, alpha/1

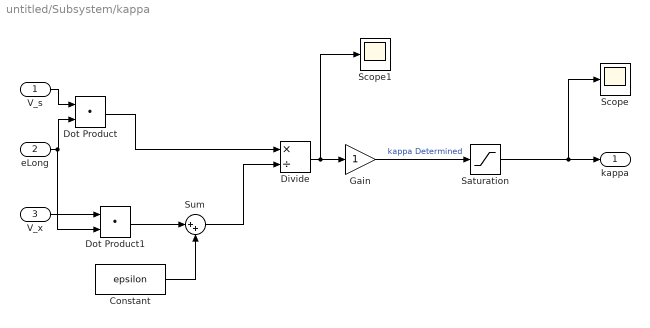
== system untitled/Subsystem/kappa ==
  V_s : Inport
  eLong : Inport  Port=2
  V_x : Inport  Port=3
  Constant : Constant  Value=epsilon
  Divide : Product  Inputs=*/
  Dot Product : DotProduct  InputSameDT=on  OutDataTypeStr=Inherit: Inherit via internal rule
  Dot Product1 : DotProduct  InputSameDT=on  OutDataTypeStr=Inherit: Inherit via internal rule
  Gain : Gain
  Saturation : Saturate  UpperLimit=0  LowerLimit=-1e0
  Scope : Scope
  Scope1 : Scope
  Sum : Sum  Inputs=|++
  kappa : Outport
  wires:
  V_s/1 -> Dot Product/1
  eLong/1 -> Dot Product1/2, Dot Product/2
  Dot Product/1 -> Divide/1
  V_x/1 -> Dot Product1/1
  Divide/1 -> Scope1/1, Gain/1
  Gain/1 -> Saturation/1  "kappa Determined"
  Dot Product1/1 -> Sum/1
  Constant/1 -> Sum/2
  Saturation/1 -> Scope/1, kappa/1
  Sum/1 -> Divide/2
